simulink model "test_quad_control_attached_real_vehicles_COMM_ONLY"  (R2019b)
settings: Solver=FixedStepAuto  StartTime=0.0  StopTime=30  FixedStep=0.01  RelTol=1e-3  EnableMultiTasking=on
InitFcn:
  | global clientID;
  | clientID=-1;
libraries: dspindex x2, simulink x1
settings Model: SimulationMode=external  EnablePacing=on  Creator=Kleber Cabral  LastModifiedBy=Kleber Cabral
settings DataIOCC: SaveFormat=Array  ReturnWorkspaceOutputs=off
settings DebuggingCC: SolverPrmCheckMsg=warning  SFUnexpectedBacktrackingDiag=warning  SFNoUnconditionalDefaultTransitionDiag=warning  ArithmeticOperatorsInVariantConditions=warning
settings HardwareCC: ProdBitPerLong=64  ProdHWDeviceType=Intel->x86-64 (Mac OS X)
settings ModelReferenceCC: PropagateSignalLabelsOutOfModel=off
settings SFSimCC: SimUseLocalCustomCode=off  CustomCodeUndefinedFunction=UseInterfaceOnly
settings RTWCC: Description=Simulink Desktop Real-Time  SystemTargetFile=sldrt.tlc  TemplateMakefile=sldrt.tmf  RTWUseLocalCustomCode=off  RTWCompilerOptimization=on
settings CodeAppCC: MaxIdLength=95  StateflowObjectComments=on
settings SimulinkDesktopRealTimeCC: TargetPreCompLibLocation=/Applications/MATLAB_R2019b.app/toolbox/sldrt/lib/maci64  TargetLangStandard=C89/C90 (ANSI)  PreserveStateflowLocalDataDimensions=off
settings ConfigComp: CovMetricSettings=dw  CovHtmlReporting=on  CovSaveCumulativeToWorkspaceVar=on  CovSaveSingleToWorkspaceVar=on  CovExternalEMLEnable=off  CovSFcnEnable=off

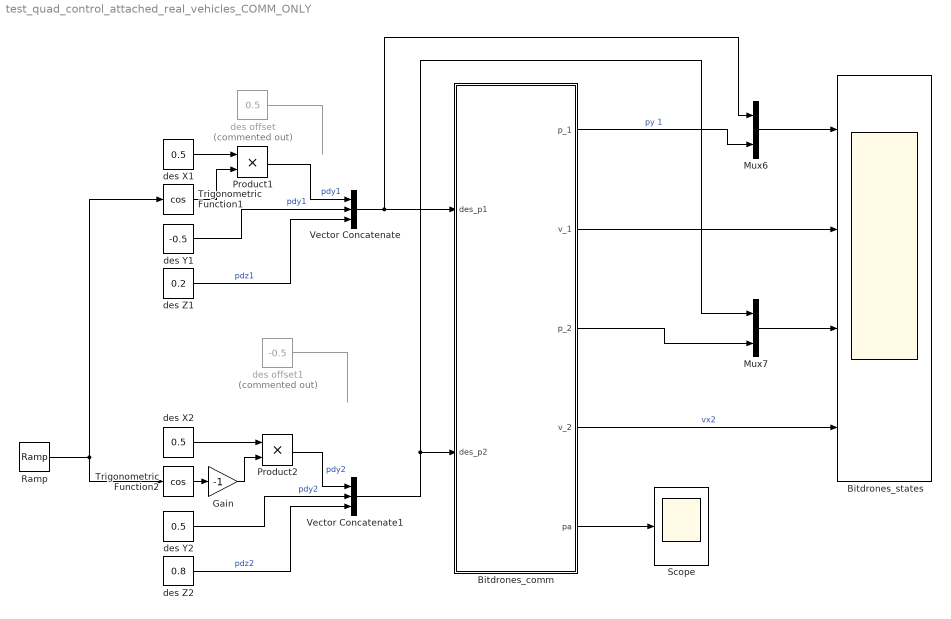
== system test_quad_control_attached_real_vehicles_COMM_ONLY ==
  Bitdrones_comm : Subsystem
  Bitdrones_states : Scope  NumInputPorts=4
  Gain : Gain  Gain=-1
  Mux6 : Mux  Inputs=2
  Mux7 : Mux  Inputs=2
  Product1 : Product
  Product2 : Product
  Ramp : simulink/Sources/Ramp  slope=0.2  start=0  InitialOutput=0
  Scope : Scope
  Trigonometric Function1 : Trigonometry  Operator=cos
  Trigonometric Function2 : Trigonometry  Operator=cos
  Vector Concatenate : Concatenate  NumInputs=3
  Vector Concatenate1 : Concatenate  NumInputs=3
  des X1 : Constant  Value=0.5
  des X2 : Constant  Value=0.5
  des Y1 : Constant  Value=-0.5  VectorParams1D=off
  des Y2 : Constant  Value=0.5  VectorParams1D=off
  des Z1 : Constant  Value=0.2
  des Z2 : Constant  Value=0.8
  des offset : Constant  Commented=on  Value=0.5
  des offset1 : Constant  Commented=on  Value=-0.5
  wires:
  Bitdrones_comm/5(pa) -> Scope/1
  Ramp/1 -> Trigonometric Function1/1, Trigonometric Function2/1
  Trigonometric Function1/1 -> Product1/2
  des X1/1 -> Product1/1
  Vector Concatenate/1 -> Bitdrones_comm/1(des_p1), Mux6/1
  des Y1/1 -> Vector Concatenate/2  "pdy1"
  des Z1/1 -> Vector Concatenate/3  "pdz1"
  des Z2/1 -> Vector Concatenate1/3  "pdz2"
  des Y2/1 -> Vector Concatenate1/2  "pdy2"
  des X2/1 -> Product2/1
  Gain/1 -> Product2/2
  Vector Concatenate1/1 -> Bitdrones_comm/2(des_p2), Mux7/1
  Mux6/1 -> Bitdrones_states/1
  Mux7/1 -> Bitdrones_states/3
  Trigonometric Function2/1 -> Gain/1
  Product1/1 -> Vector Concatenate/1  "pdy1"
  des offset/1 -> ?
  Product2/1 -> Vector Concatenate1/1  "pdy2"
  des offset1/1 -> ?
  Bitdrones_comm/1(p_1) -> Mux6/2  "py 1"
  Bitdrones_comm/2(v_1) -> Bitdrones_states/2
  Bitdrones_comm/3(p_2) -> Mux7/2
  Bitdrones_comm/4(v_2) -> Bitdrones_states/4  "vx2"

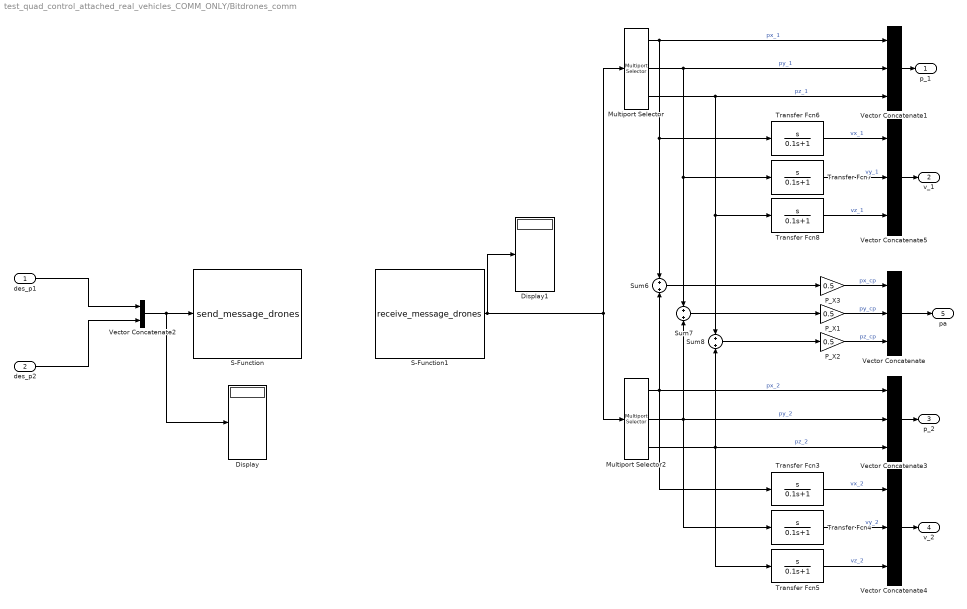
== system test_quad_control_attached_real_vehicles_COMM_ONLY/Bitdrones_comm ==
  des_p1 : Inport
  des_p2 : Inport  Port=2
  Display : Display
      settings: Decimation=3
  Display1 : Display
      settings: Decimation=3
  Multiport Selector : dspindex/Multiport Selector  rowsOrCols=Rows  idxCellArray={1,2,3}  idxErrMode=Clip Index
  Multiport Selector2 : dspindex/Multiport Selector  rowsOrCols=Rows  idxCellArray={4,5,6}  idxErrMode=Clip Index
  P_X1 : Gain  Gain=0.5
  P_X2 : Gain  Gain=0.5
  P_X3 : Gain  Gain=0.5
  S-Function : S-Function  FunctionName=send_message_drones  SFunctionDeploymentMode=off  EnableBusSupport=off
  S-Function1 : S-Function  FunctionName=receive_message_drones  SFunctionDeploymentMode=off  EnableBusSupport=off
  Sum6 : Sum  Inputs=+|+
  Sum7 : Sum  Inputs=+|+
  Sum8 : Sum  Inputs=+|+
  Transfer Fcn{3..8} (6 alike) : TransferFcn  Numerator=[1 0]  Denominator=[0.1 1]
  Vector Concatenate{,1,3..5} (5 alike) : Concatenate  NumInputs=3
  Vector Concatenate2 : Concatenate
  p_1 : Outport
  v_1 : Outport  Port=2
  p_2 : Outport  Port=3
  v_2 : Outport  Port=4
  pa : Outport  Port=5
  wires:
  Multiport Selector/1 -> Vector Concatenate1/1, Transfer Fcn6/1, Sum6/1  "px_1"
  Multiport Selector/2 -> Vector Concatenate1/2, Transfer Fcn7/1, Sum7/1  "py_1"
  Multiport Selector/3 -> Vector Concatenate1/3, Transfer Fcn8/1, Sum8/1  "pz_1"
  Sum6/1 -> P_X3/1
  Multiport Selector2/1 -> Vector Concatenate3/1, Transfer Fcn3/1, Sum6/2  "px_2"
  Multiport Selector2/2 -> Vector Concatenate3/2, Transfer Fcn4/1, Sum7/2  "py_2"
  Multiport Selector2/3 -> Transfer Fcn5/1, Vector Concatenate3/3, Sum8/2  "pz_2"
  Sum7/1 -> P_X1/1
  Sum8/1 -> P_X2/1
  S-Function1/1 -> Display1/1, Multiport Selector/1, Multiport Selector2/1
  Vector Concatenate2/1 -> Display/1, S-Function/1
  des_p2/1 -> Vector Concatenate2/2
  des_p1/1 -> Vector Concatenate2/1
  Transfer Fcn4/1 -> Vector Concatenate4/2  "vy_2"
  Transfer Fcn5/1 -> Vector Concatenate4/3  "vz_2"
  P_X1/1 -> Vector Concatenate/2  "py_cp"
  Vector Concatenate/1 -> pa/1
  P_X3/1 -> Vector Concatenate/1  "px_cp"
  P_X2/1 -> Vector Concatenate/3  "pz_cp"
  Vector Concatenate1/1 -> p_1/1
  Vector Concatenate3/1 -> p_2/1
  Vector Concatenate4/1 -> v_2/1
  Transfer Fcn3/1 -> Vector Concatenate4/1  "vx_2"
  Transfer Fcn6/1 -> Vector Concatenate5/1  "vx_1"
  Vector Concatenate5/1 -> v_1/1
  Transfer Fcn8/1 -> Vector Concatenate5/3  "vz_1"
  Transfer Fcn7/1 -> Vector Concatenate5/2  "vy_1"
